simulink model "active_vehicle_ESP_Control"  (R2020a)
settings: Solver=ode4  StartTime=0.0  StopTime=inf  FixedStep=1e-3  RelTol=1e-3
InitFcn:
  | clear mex
model workspace (MAT data in the model file):
  inChnlList : object (value not decoded)
  inChnlListInternal : object (value not decoded)
  outChnlList : object (value not decoded)
  outChnlListInternal : object (value not decoded)
undefined symbols (not defined in the file or in its folder): DiscIntNeverNeededParam, vicrt_initcallback, vicrt_initmexcallback, vicrt_inputfile, vicrt_simulationmanager
libraries: simulink x1
(part 5 of 6)

== system active_vehicle_ESP_Control/Driveline/Engine/Engine Maps/Rpm control/idle control ==
  engine omega : Inport
  idle speed : Inport  Port=2
  Add2 : Sum  Inputs=+-  OutDataTypeStr=Inherit: Same as first input
  Gain : Gain  Gain=100*0.005/((2*pi/60))  OutDataTypeStr=Inherit: Same as input  ParamDataTypeStr=Inherit: Same as input
  Switch : Switch  Criteria=u2 > Threshold
  Unary Minus : UnaryMinus
  zero : Constant  Value=0
  rpm_idle_contrlol : Outport
  wires:
  engine omega/1 -> Add2/1
  idle speed/1 -> Add2/2
  Add2/1 -> Switch/2, Unary Minus/1
  zero/1 -> Switch/1
  Unary Minus/1 -> Gain/1
  Gain/1 -> Switch/3
  Switch/1 -> rpm_idle_contrlol/1

== system active_vehicle_ESP_Control/Vehicle/VI-CarRealTime/Input_Bus/Inputs/ABS ==
  ABS_threshold_def_val : Constant  Value=0
  BCABS : BusCreator  Inputs=2
  Internal_ABS_Activity_def_val : Constant
  ABS : Outport
  wires:
  BCABS/1 -> ABS/1  "ABS"
  Internal_ABS_Activity_def_val/1 -> BCABS/1  "Internal_ABS_Activity"
  ABS_threshold_def_val/1 -> BCABS/2  "ABS_threshold"

== system active_vehicle_ESP_Control/Vehicle/VI-CarRealTime/Input_Bus/Inputs/Aerodynamic ==
  BCAerodynamic : BusCreator  Inputs=16
  fx_center_def_val : Constant  Value=0
  fx_central_scaling_def_val : Constant
  fx_front_def_val : Constant  Value=0
  fx_rear_def_val : Constant  Value=0
  fy_center_def_val : Constant  Value=0
  fy_front_def_val : Constant  Value=0
  fy_rear_def_val : Constant  Value=0
  fz_center_def_val : Constant  Value=0
  fz_front_def_val : Constant  Value=0
  fz_front_scaling_def_val : Constant
  fz_rear_def_val : Constant  Value=0
  fz_rear_scaling_def_val : Constant
  mx_def_val : Constant  Value=0
  my_def_val : Constant  Value=0
  my_scaling_def_val : Constant
  mz_def_val : Constant  Value=0
  Aerodynamic : Outport
  wires:
  BCAerodynamic/1 -> Aerodynamic/1  "Aerodynamic"
  my_scaling_def_val/1 -> BCAerodynamic/1  "my_scaling"
  fx_central_scaling_def_val/1 -> BCAerodynamic/2  "fx_central_scaling"
  fz_front_scaling_def_val/1 -> BCAerodynamic/3  "fz_front_scaling"
  fz_rear_scaling_def_val/1 -> BCAerodynamic/4  "fz_rear_scaling"
  fx_front_def_val/1 -> BCAerodynamic/5  "fx_front"
  fy_front_def_val/1 -> BCAerodynamic/6  "fy_front"
  fz_front_def_val/1 -> BCAerodynamic/7  "fz_front"
  fx_rear_def_val/1 -> BCAerodynamic/8  "fx_rear"
  fy_rear_def_val/1 -> BCAerodynamic/9  "fy_rear"
  fz_rear_def_val/1 -> BCAerodynamic/10  "fz_rear"
  fx_center_def_val/1 -> BCAerodynamic/11  "fx_center"
  fy_center_def_val/1 -> BCAerodynamic/12  "fy_center"
  fz_center_def_val/1 -> BCAerodynamic/13  "fz_center"
  mx_def_val/1 -> BCAerodynamic/14  "mx"
  my_def_val/1 -> BCAerodynamic/15  "my"
  mz_def_val/1 -> BCAerodynamic/16  "mz"

== system active_vehicle_ESP_Control/Vehicle/VI-CarRealTime/Input_Bus/Inputs/Antiroll_Bar ==
  BCAntiroll_Bar : BusCreator  Inputs=2
  activity_flag : Subsystem
  force : Subsystem
  Antiroll_Bar : Outport
  wires:
  BCAntiroll_Bar/1 -> Antiroll_Bar/1  "Antiroll_Bar"
  activity_flag/1(activity_flag) -> BCAntiroll_Bar/1  "activity_flag"
  force/1(force) -> BCAntiroll_Bar/2  "force"

== system active_vehicle_ESP_Control/Vehicle/VI-CarRealTime/Input_Bus/Inputs/Auxiliary_vertical ==
  BCAuxiliary_vertical : BusCreator  Inputs=2
  activity_flag : Subsystem
  force : Subsystem
  Auxiliary_vertical : Outport
  wires:
  BCAuxiliary_vertical/1 -> Auxiliary_vertical/1  "Auxiliary_vertical"
  force/1(force) -> BCAuxiliary_vertical/1  "force"
  activity_flag/1(activity_flag) -> BCAuxiliary_vertical/2  "activity_flag"

== system active_vehicle_ESP_Control/Vehicle/VI-CarRealTime/Input_Bus/Inputs/Brake_System ==
  BCBrake_System : BusCreator  Inputs=5
  brk_mmag_sign : Subsystem
  brk_mmag_unsign : Subsystem
  brk_mu : Subsystem
  brk_pres : Subsystem
  brk_pres_gain : Subsystem
  Brake_System : Outport
  wires:
  BCBrake_System/1 -> Brake_System/1  "Brake_System"
  brk_mmag_sign/1(brk_mmag_sign) -> BCBrake_System/1  "brk_mmag_sign"
  brk_mmag_unsign/1(brk_mmag_unsign) -> BCBrake_System/2  "brk_mmag_unsign"
  brk_pres/1(brk_pres) -> BCBrake_System/3  "brk_pres"
  brk_pres_gain/1(brk_pres_gain) -> BCBrake_System/4  "brk_pres_gain"
  brk_mu/1(brk_mu) -> BCBrake_System/5  "brk_mu"

== system active_vehicle_ESP_Control/Vehicle/VI-CarRealTime/Input_Bus/Inputs/Brake_System_General ==
  BCBrake_System_General : BusCreator  Inputs=2
  brk_bias_front_def_val : Constant  Value=0
  brk_mast_cyl_pres_def_val : Constant  Value=0
  Brake_System_General : Outport
  wires:
  BCBrake_System_General/1 -> Brake_System_General/1  "Brake_System_General"
  brk_mast_cyl_pres_def_val/1 -> BCBrake_System_General/1  "brk_mast_cyl_pres"
  brk_bias_front_def_val/1 -> BCBrake_System_General/2  "brk_bias_front"

== system active_vehicle_ESP_Control/Vehicle/VI-CarRealTime/Input_Bus/Inputs/Clutch ==
  BCClutch : BusCreator  Inputs=6
  clutch_trq_def_val : Constant  Value=0
  efficiency_def_val : Constant
  gearbox_inputshaft_torque_def_val : Constant  Value=0
  inputplate_alpha_def_val : Constant  Value=-9999999
  inputplate_angle_def_val : Constant  Value=-9999999
  inputplate_omega_def_val : Constant  Value=-9999999
  Clutch : Outport
  wires:
  BCClutch/1 -> Clutch/1  "Clutch"
  clutch_trq_def_val/1 -> BCClutch/1  "clutch_trq"
  gearbox_inputshaft_torque_def_val/1 -> BCClutch/2  "gearbox_inputshaft_torque"
  inputplate_angle_def_val/1 -> BCClutch/3  "inputplate_angle"
  inputplate_omega_def_val/1 -> BCClutch/4  "inputplate_omega"
  inputplate_alpha_def_val/1 -> BCClutch/5  "inputplate_alpha"
  efficiency_def_val/1 -> BCClutch/6  "efficiency"

== system active_vehicle_ESP_Control/Vehicle/VI-CarRealTime/Input_Bus/Inputs/Differential_Central ==
  BCDifferential_Central : BusCreator  Inputs=6
  diff_front_inputshaft_torque_def_val : Constant  Value=0
  diff_rear_inputshaft_torque_def_val : Constant  Value=0
  efficiency_def_val : Constant
  gearbox_outputshaft_alpha_def_val : Constant  Value=0
  gearbox_outputshaft_angle_def_val : Constant  Value=0
  gearbox_outputshaft_omega_def_val : Constant  Value=0
  Differential_Central : Outport
  wires:
  BCDifferential_Central/1 -> Differential_Central/1  "Differential_Central"
  efficiency_def_val/1 -> BCDifferential_Central/1  "efficiency"
  diff_front_inputshaft_torque_def_val/1 -> BCDifferential_Central/2  "diff_front_inputshaft_torque"
  diff_rear_inputshaft_torque_def_val/1 -> BCDifferential_Central/3  "diff_rear_inputshaft_torque"
  gearbox_outputshaft_angle_def_val/1 -> BCDifferential_Central/4  "gearbox_outputshaft_angle"
  gearbox_outputshaft_omega_def_val/1 -> BCDifferential_Central/5  "gearbox_outputshaft_omega"
  gearbox_outputshaft_alpha_def_val/1 -> BCDifferential_Central/6  "gearbox_outputshaft_alpha"

== system active_vehicle_ESP_Control/Vehicle/VI-CarRealTime/Input_Bus/Inputs/Differential_Front ==
  BCDifferential_Front : BusCreator  Inputs=6
  diff_central_front_outputshaft_alpha_def_val : Constant  Value=0
  diff_central_front_outputshaft_angle_def_val : Constant  Value=0
  diff_central_front_outputshaft_omega_def_val : Constant  Value=0
  efficiency_def_val : Constant
  wheel_front_left_torque_def_val : Constant  Value=0
  wheel_front_right_torque_def_val : Constant  Value=0
  Differential_Front : Outport
  wires:
  BCDifferential_Front/1 -> Differential_Front/1  "Differential_Front"
  efficiency_def_val/1 -> BCDifferential_Front/1  "efficiency"
  wheel_front_left_torque_def_val/1 -> BCDifferential_Front/2  "wheel_front_left_torque"
  wheel_front_right_torque_def_val/1 -> BCDifferential_Front/3  "wheel_front_right_torque"
  diff_central_front_outputshaft_angle_def_val/1 -> BCDifferential_Front/4  "diff_central_front_outputshaft_angle"
  diff_central_front_outputshaft_omega_def_val/1 -> BCDifferential_Front/5  "diff_central_front_outputshaft_omega"
  diff_central_front_outputshaft_alpha_def_val/1 -> BCDifferential_Front/6  "diff_central_front_outputshaft_alpha"

== system active_vehicle_ESP_Control/Vehicle/VI-CarRealTime/Input_Bus/Inputs/Differential_Rear ==
  BCDifferential_Rear : BusCreator  Inputs=6
  diff_central_rear_outputshaft_alpha_def_val : Constant  Value=0
  diff_central_rear_outputshaft_angle_def_val : Constant  Value=0
  diff_central_rear_outputshaft_omega_def_val : Constant  Value=0
  efficiency_def_val : Constant
  wheel_rear_left_torque_def_val : Constant  Value=0
  wheel_rear_right_torque_def_val : Constant  Value=0
  Differential_Rear : Outport
  wires:
  BCDifferential_Rear/1 -> Differential_Rear/1  "Differential_Rear"
  efficiency_def_val/1 -> BCDifferential_Rear/1  "efficiency"
  wheel_rear_left_torque_def_val/1 -> BCDifferential_Rear/2  "wheel_rear_left_torque"
  wheel_rear_right_torque_def_val/1 -> BCDifferential_Rear/3  "wheel_rear_right_torque"
  diff_central_rear_outputshaft_angle_def_val/1 -> BCDifferential_Rear/4  "diff_central_rear_outputshaft_angle"
  diff_central_rear_outputshaft_omega_def_val/1 -> BCDifferential_Rear/5  "diff_central_rear_outputshaft_omega"
  diff_central_rear_outputshaft_alpha_def_val/1 -> BCDifferential_Rear/6  "diff_central_rear_outputshaft_alpha"

== system active_vehicle_ESP_Control/Vehicle/VI-CarRealTime/Input_Bus/Inputs/Driver_Demands ==
  BCDriver_Demands : BusCreator  Inputs=14
  brake_def_val : Constant  Value=0
  clutch_def_val : Constant  Value=0
  gear_def_val : Constant  Value=0
  rack_displacement_def_val : Constant  Value=0
  str_swa_def_val : Constant  Value=0
  target_acc_def_val : Constant  Value=0
  target_speed_def_val : Constant  Value=0
  throttle_def_val : Constant  Value=0
  user_input_braking_def_val : Constant  Value=0
  user_input_clutch_def_val : Constant  Value=0
  user_input_gear_def_val : Constant  Value=0
  user_input_steering_def_val : Constant  Value=0
  user_input_throttle_def_val : Constant  Value=0
  user_maneuver_ID_def_val : Constant  Value=0
  Driver_Demands : Outport
  wires:
  BCDriver_Demands/1 -> Driver_Demands/1  "Driver_Demands"
  str_swa_def_val/1 -> BCDriver_Demands/1  "str_swa"
  rack_displacement_def_val/1 -> BCDriver_Demands/2  "rack_displacement"
  throttle_def_val/1 -> BCDriver_Demands/3  "throttle"
  gear_def_val/1 -> BCDriver_Demands/4  "gear"
  clutch_def_val/1 -> BCDriver_Demands/5  "clutch"
  brake_def_val/1 -> BCDriver_Demands/6  "brake"
  target_speed_def_val/1 -> BCDriver_Demands/7  "target_speed"
  target_acc_def_val/1 -> BCDriver_Demands/8  "target_acc"
  user_maneuver_ID_def_val/1 -> BCDriver_Demands/9  "user_maneuver_ID"
  user_input_steering_def_val/1 -> BCDriver_Demands/10  "user_input_steering"
  user_input_throttle_def_val/1 -> BCDriver_Demands/11  "user_input_throttle"
  user_input_braking_def_val/1 -> BCDriver_Demands/12  "user_input_braking"
  user_input_gear_def_val/1 -> BCDriver_Demands/13  "user_input_gear"
  user_input_clutch_def_val/1 -> BCDriver_Demands/14  "user_input_clutch"

== system active_vehicle_ESP_Control/Vehicle/VI-CarRealTime/Input_Bus/Inputs/Engine ==
  BCEngine : BusCreator  Inputs=10
  clutch_inputplate_torque_def_val : Constant  Value=0
  control_mode_def_val : Constant
  efficiency_def_val : Constant
  engine_max_trq_def_val : Constant  Value=0
  engine_min_trq_def_val : Constant  Value=0
  engine_omega_def_val : Constant  Value=0
  engine_trq_def_val : Constant  Value=0
  non_termic_engine_trq_def_val : Constant  Value=0
  throttle_offset_def_val : Constant  Value=0
  throttle_scaling_def_val : Constant
  Engine : Outport
  wires:
  BCEngine/1 -> Engine/1  "Engine"
  engine_omega_def_val/1 -> BCEngine/1  "engine_omega"
  engine_max_trq_def_val/1 -> BCEngine/2  "engine_max_trq"
  engine_min_trq_def_val/1 -> BCEngine/3  "engine_min_trq"
  engine_trq_def_val/1 -> BCEngine/4  "engine_trq"
  clutch_inputplate_torque_def_val/1 -> BCEngine/5  "clutch_inputplate_torque"
  non_termic_engine_trq_def_val/1 -> BCEngine/6  "non_termic_engine_trq"
  efficiency_def_val/1 -> BCEngine/7  "efficiency"
  throttle_scaling_def_val/1 -> BCEngine/8  "throttle_scaling"
  control_mode_def_val/1 -> BCEngine/9  "control_mode"
  throttle_offset_def_val/1 -> BCEngine/10  "throttle_offset"

== system active_vehicle_ESP_Control/Vehicle/VI-CarRealTime/Input_Bus/Inputs/Ext_Body ==
  BCExt_Body : BusCreator  Inputs=2
  force : Subsystem
  moment : Subsystem
  Ext_Body : Outport
  wires:
  BCExt_Body/1 -> Ext_Body/1  "Ext_Body"
  force/1(force) -> BCExt_Body/1  "force"
  moment/1(moment) -> BCExt_Body/2  "moment"

== system active_vehicle_ESP_Control/Vehicle/VI-CarRealTime/Input_Bus/Inputs/Ext_Ground ==
  BCExt_Ground : BusCreator  Inputs=2
  force : Subsystem
  moment : Subsystem
  Ext_Ground : Outport
  wires:
  BCExt_Ground/1 -> Ext_Ground/1  "Ext_Ground"
  force/1(force) -> BCExt_Ground/1  "force"
  moment/1(moment) -> BCExt_Ground/2  "moment"

== system active_vehicle_ESP_Control/Vehicle/VI-CarRealTime/Input_Bus/Inputs/Ext_Tracking ==
  BCExt_Tracking : BusCreator  Inputs=2
  force : Subsystem
  moment : Subsystem
  Ext_Tracking : Outport
  wires:
  BCExt_Tracking/1 -> Ext_Tracking/1  "Ext_Tracking"
  force/1(force) -> BCExt_Tracking/1  "force"
  moment/1(moment) -> BCExt_Tracking/2  "moment"

== system active_vehicle_ESP_Control/Vehicle/VI-CarRealTime/Input_Bus/Inputs/Friction ==
  BCFriction : BusCreator  Inputs=1
  tire_mu : Subsystem
  Friction : Outport
  wires:
  BCFriction/1 -> Friction/1  "Friction"
  tire_mu/1(tire_mu) -> BCFriction/1  "tire_mu"

== system active_vehicle_ESP_Control/Vehicle/VI-CarRealTime/Input_Bus/Inputs/GearBox ==
  BCGearBox : BusCreator  Inputs=7
  automatic_gearbox_shifting_mode_def_val : Constant  Value=-9999999
  clutch_outputplate_alpha_def_val : Constant  Value=-9999999
  clutch_outputplate_angle_def_val : Constant  Value=-9999999
  clutch_outputplate_omega_def_val : Constant  Value=-9999999
  diff_central_inputshaft_torque_def_val : Constant  Value=0
  efficiency_def_val : Constant
  transmission_ratio_def_val : Constant  Value=0
  GearBox : Outport
  wires:
  BCGearBox/1 -> GearBox/1  "GearBox"
  efficiency_def_val/1 -> BCGearBox/1  "efficiency"
  transmission_ratio_def_val/1 -> BCGearBox/2  "transmission_ratio"
  diff_central_inputshaft_torque_def_val/1 -> BCGearBox/3  "diff_central_inputshaft_torque"
  clutch_outputplate_angle_def_val/1 -> BCGearBox/4  "clutch_outputplate_angle"
  clutch_outputplate_omega_def_val/1 -> BCGearBox/5  "clutch_outputplate_omega"
  clutch_outputplate_alpha_def_val/1 -> BCGearBox/6  "clutch_outputplate_alpha"
  automatic_gearbox_shifting_mode_def_val/1 -> BCGearBox/7  "automatic_gearbox_shifting_mode"

== system active_vehicle_ESP_Control/Vehicle/VI-CarRealTime/Input_Bus/Inputs/Generic_Engine_to_Central_Differential ==
  BCGeneric_Engine_to_Central_Differential : BusCreator  Inputs=10
  control_mode_def_val : Constant
  efficiency_def_val : Constant
  engine_max_torque_def_val : Constant  Value=0
  engine_min_torque_def_val : Constant  Value=0
  engine_torque_def_val : Constant  Value=0
  regeneration_factor_def_val : Constant
  reverse_mode_def_val : Constant  Value=0
  throttle_offset_def_val : Constant  Value=0
  throttle_scaling_def_val : Constant
  transmission_ratio_def_val : Constant
  Generic_Engine_to_Central_Differential : Outport
  wires:
  BCGeneric_Engine_to_Central_Differential/1 -> Generic_Engine_to_Central_Differential/1  "Generic_Engine_to_Central_Differential"
  transmission_ratio_def_val/1 -> BCGeneric_Engine_to_Central_Differential/1  "transmission_ratio"
  reverse_mode_def_val/1 -> BCGeneric_Engine_to_Central_Differential/2  "reverse_mode"
  regeneration_factor_def_val/1 -> BCGeneric_Engine_to_Central_Differential/3  "regeneration_factor"
  throttle_scaling_def_val/1 -> BCGeneric_Engine_to_Central_Differential/4  "throttle_scaling"
  control_mode_def_val/1 -> BCGeneric_Engine_to_Central_Differential/5  "control_mode"
  throttle_offset_def_val/1 -> BCGeneric_Engine_to_Central_Differential/6  "throttle_offset"
  efficiency_def_val/1 -> BCGeneric_Engine_to_Central_Differential/7  "efficiency"
  engine_torque_def_val/1 -> BCGeneric_Engine_to_Central_Differential/8  "engine_torque"
  engine_max_torque_def_val/1 -> BCGeneric_Engine_to_Central_Differential/9  "engine_max_torque"
  engine_min_torque_def_val/1 -> BCGeneric_Engine_to_Central_Differential/10  "engine_min_torque"

== system active_vehicle_ESP_Control/Vehicle/VI-CarRealTime/Input_Bus/Inputs/Generic_Engine_to_Clutch ==
  BCGeneric_Engine_to_Clutch : BusCreator  Inputs=9
  control_mode_def_val : Constant
  efficiency_def_val : Constant
  engine_max_torque_def_val : Constant  Value=0
  engine_min_torque_def_val : Constant  Value=0
  engine_torque_def_val : Constant  Value=0
  regeneration_factor_def_val : Constant
  throttle_offset_def_val : Constant  Value=0
  throttle_scaling_def_val : Constant
  transmission_ratio_def_val : Constant
  Generic_Engine_to_Clutch : Outport
  wires:
  BCGeneric_Engine_to_Clutch/1 -> Generic_Engine_to_Clutch/1  "Generic_Engine_to_Clutch"
  transmission_ratio_def_val/1 -> BCGeneric_Engine_to_Clutch/1  "transmission_ratio"
  regeneration_factor_def_val/1 -> BCGeneric_Engine_to_Clutch/2  "regeneration_factor"
  throttle_scaling_def_val/1 -> BCGeneric_Engine_to_Clutch/3  "throttle_scaling"
  control_mode_def_val/1 -> BCGeneric_Engine_to_Clutch/4  "control_mode"
  throttle_offset_def_val/1 -> BCGeneric_Engine_to_Clutch/5  "throttle_offset"
  efficiency_def_val/1 -> BCGeneric_Engine_to_Clutch/6  "efficiency"
  engine_torque_def_val/1 -> BCGeneric_Engine_to_Clutch/7  "engine_torque"
  engine_max_torque_def_val/1 -> BCGeneric_Engine_to_Clutch/8  "engine_max_torque"
  engine_min_torque_def_val/1 -> BCGeneric_Engine_to_Clutch/9  "engine_min_torque"

== system active_vehicle_ESP_Control/Vehicle/VI-CarRealTime/Input_Bus/Inputs/Generic_Engine_to_Front_Differential ==
  BCGeneric_Engine_to_Front_Differential : BusCreator  Inputs=10
  control_mode_def_val : Constant
  efficiency_def_val : Constant
  engine_max_torque_def_val : Constant  Value=0
  engine_min_torque_def_val : Constant  Value=0
  engine_torque_def_val : Constant  Value=0
  regeneration_factor_def_val : Constant
  reverse_mode_def_val : Constant  Value=0
  throttle_offset_def_val : Constant  Value=0
  throttle_scaling_def_val : Constant
  transmission_ratio_def_val : Constant
  Generic_Engine_to_Front_Differential : Outport
  wires:
  BCGeneric_Engine_to_Front_Differential/1 -> Generic_Engine_to_Front_Differential/1  "Generic_Engine_to_Front_Differential"
  transmission_ratio_def_val/1 -> BCGeneric_Engine_to_Front_Differential/1  "transmission_ratio"
  reverse_mode_def_val/1 -> BCGeneric_Engine_to_Front_Differential/2  "reverse_mode"
  regeneration_factor_def_val/1 -> BCGeneric_Engine_to_Front_Differential/3  "regeneration_factor"
  throttle_scaling_def_val/1 -> BCGeneric_Engine_to_Front_Differential/4  "throttle_scaling"
  control_mode_def_val/1 -> BCGeneric_Engine_to_Front_Differential/5  "control_mode"
  throttle_offset_def_val/1 -> BCGeneric_Engine_to_Front_Differential/6  "throttle_offset"
  efficiency_def_val/1 -> BCGeneric_Engine_to_Front_Differential/7  "efficiency"
  engine_torque_def_val/1 -> BCGeneric_Engine_to_Front_Differential/8  "engine_torque"
  engine_max_torque_def_val/1 -> BCGeneric_Engine_to_Front_Differential/9  "engine_max_torque"
  engine_min_torque_def_val/1 -> BCGeneric_Engine_to_Front_Differential/10  "engine_min_torque"

== system active_vehicle_ESP_Control/Vehicle/VI-CarRealTime/Input_Bus/Inputs/Generic_Engine_to_Front_Left_Wheel ==
  BCGeneric_Engine_to_Front_Left_Wheel : BusCreator  Inputs=10
  control_mode_def_val : Constant
  efficiency_def_val : Constant
  engine_max_torque_def_val : Constant  Value=0
  engine_min_torque_def_val : Constant  Value=0
  engine_torque_def_val : Constant  Value=0
  regeneration_factor_def_val : Constant
  reverse_mode_def_val : Constant  Value=0
  throttle_offset_def_val : Constant  Value=0
  throttle_scaling_def_val : Constant
  transmission_ratio_def_val : Constant
  Generic_Engine_to_Front_Left_Wheel : Outport
  wires:
  BCGeneric_Engine_to_Front_Left_Wheel/1 -> Generic_Engine_to_Front_Left_Wheel/1  "Generic_Engine_to_Front_Left_Wheel"
  transmission_ratio_def_val/1 -> BCGeneric_Engine_to_Front_Left_Wheel/1  "transmission_ratio"
  reverse_mode_def_val/1 -> BCGeneric_Engine_to_Front_Left_Wheel/2  "reverse_mode"
  regeneration_factor_def_val/1 -> BCGeneric_Engine_to_Front_Left_Wheel/3  "regeneration_factor"
  throttle_scaling_def_val/1 -> BCGeneric_Engine_to_Front_Left_Wheel/4  "throttle_scaling"
  control_mode_def_val/1 -> BCGeneric_Engine_to_Front_Left_Wheel/5  "control_mode"
  throttle_offset_def_val/1 -> BCGeneric_Engine_to_Front_Left_Wheel/6  "throttle_offset"
  efficiency_def_val/1 -> BCGeneric_Engine_to_Front_Left_Wheel/7  "efficiency"
  engine_torque_def_val/1 -> BCGeneric_Engine_to_Front_Left_Wheel/8  "engine_torque"
  engine_max_torque_def_val/1 -> BCGeneric_Engine_to_Front_Left_Wheel/9  "engine_max_torque"
  engine_min_torque_def_val/1 -> BCGeneric_Engine_to_Front_Left_Wheel/10  "engine_min_torque"

== system active_vehicle_ESP_Control/Vehicle/VI-CarRealTime/Input_Bus/Inputs/Generic_Engine_to_Front_Right_Wheel ==
  BCGeneric_Engine_to_Front_Right_Wheel : BusCreator  Inputs=10
  control_mode_def_val : Constant
  efficiency_def_val : Constant
  engine_max_torque_def_val : Constant  Value=0
  engine_min_torque_def_val : Constant  Value=0
  engine_torque_def_val : Constant  Value=0
  regeneration_factor_def_val : Constant
  reverse_mode_def_val : Constant  Value=0
  throttle_offset_def_val : Constant  Value=0
  throttle_scaling_def_val : Constant
  transmission_ratio_def_val : Constant
  Generic_Engine_to_Front_Right_Wheel : Outport
  wires:
  BCGeneric_Engine_to_Front_Right_Wheel/1 -> Generic_Engine_to_Front_Right_Wheel/1  "Generic_Engine_to_Front_Right_Wheel"
  transmission_ratio_def_val/1 -> BCGeneric_Engine_to_Front_Right_Wheel/1  "transmission_ratio"
  reverse_mode_def_val/1 -> BCGeneric_Engine_to_Front_Right_Wheel/2  "reverse_mode"
  regeneration_factor_def_val/1 -> BCGeneric_Engine_to_Front_Right_Wheel/3  "regeneration_factor"
  throttle_scaling_def_val/1 -> BCGeneric_Engine_to_Front_Right_Wheel/4  "throttle_scaling"
  control_mode_def_val/1 -> BCGeneric_Engine_to_Front_Right_Wheel/5  "control_mode"
  throttle_offset_def_val/1 -> BCGeneric_Engine_to_Front_Right_Wheel/6  "throttle_offset"
  efficiency_def_val/1 -> BCGeneric_Engine_to_Front_Right_Wheel/7  "efficiency"
  engine_torque_def_val/1 -> BCGeneric_Engine_to_Front_Right_Wheel/8  "engine_torque"
  engine_max_torque_def_val/1 -> BCGeneric_Engine_to_Front_Right_Wheel/9  "engine_max_torque"
  engine_min_torque_def_val/1 -> BCGeneric_Engine_to_Front_Right_Wheel/10  "engine_min_torque"

== system active_vehicle_ESP_Control/Vehicle/VI-CarRealTime/Input_Bus/Inputs/Generic_Engine_to_Gearbox ==
  BCGeneric_Engine_to_Gearbox : BusCreator  Inputs=9
  control_mode_def_val : Constant
  efficiency_def_val : Constant
  engine_max_torque_def_val : Constant  Value=0
  engine_min_torque_def_val : Constant  Value=0
  engine_torque_def_val : Constant  Value=0
  regeneration_factor_def_val : Constant
  throttle_offset_def_val : Constant  Value=0
  throttle_scaling_def_val : Constant
  transmission_ratio_def_val : Constant
  Generic_Engine_to_Gearbox : Outport
  wires:
  BCGeneric_Engine_to_Gearbox/1 -> Generic_Engine_to_Gearbox/1  "Generic_Engine_to_Gearbox"
  transmission_ratio_def_val/1 -> BCGeneric_Engine_to_Gearbox/1  "transmission_ratio"
  regeneration_factor_def_val/1 -> BCGeneric_Engine_to_Gearbox/2  "regeneration_factor"
  throttle_scaling_def_val/1 -> BCGeneric_Engine_to_Gearbox/3  "throttle_scaling"
  control_mode_def_val/1 -> BCGeneric_Engine_to_Gearbox/4  "control_mode"
  throttle_offset_def_val/1 -> BCGeneric_Engine_to_Gearbox/5  "throttle_offset"
  efficiency_def_val/1 -> BCGeneric_Engine_to_Gearbox/6  "efficiency"
  engine_torque_def_val/1 -> BCGeneric_Engine_to_Gearbox/7  "engine_torque"
  engine_max_torque_def_val/1 -> BCGeneric_Engine_to_Gearbox/8  "engine_max_torque"
  engine_min_torque_def_val/1 -> BCGeneric_Engine_to_Gearbox/9  "engine_min_torque"

== system active_vehicle_ESP_Control/Vehicle/VI-CarRealTime/Input_Bus/Inputs/Generic_Engine_to_Rear_Differential ==
  BCGeneric_Engine_to_Rear_Differential : BusCreator  Inputs=10
  control_mode_def_val : Constant
  efficiency_def_val : Constant
  engine_max_torque_def_val : Constant  Value=0
  engine_min_torque_def_val : Constant  Value=0
  engine_torque_def_val : Constant  Value=0
  regeneration_factor_def_val : Constant
  reverse_mode_def_val : Constant  Value=0
  throttle_offset_def_val : Constant  Value=0
  throttle_scaling_def_val : Constant
  transmission_ratio_def_val : Constant
  Generic_Engine_to_Rear_Differential : Outport
  wires:
  BCGeneric_Engine_to_Rear_Differential/1 -> Generic_Engine_to_Rear_Differential/1  "Generic_Engine_to_Rear_Differential"
  transmission_ratio_def_val/1 -> BCGeneric_Engine_to_Rear_Differential/1  "transmission_ratio"
  reverse_mode_def_val/1 -> BCGeneric_Engine_to_Rear_Differential/2  "reverse_mode"
  regeneration_factor_def_val/1 -> BCGeneric_Engine_to_Rear_Differential/3  "regeneration_factor"
  throttle_scaling_def_val/1 -> BCGeneric_Engine_to_Rear_Differential/4  "throttle_scaling"
  control_mode_def_val/1 -> BCGeneric_Engine_to_Rear_Differential/5  "control_mode"
  throttle_offset_def_val/1 -> BCGeneric_Engine_to_Rear_Differential/6  "throttle_offset"
  efficiency_def_val/1 -> BCGeneric_Engine_to_Rear_Differential/7  "efficiency"
  engine_torque_def_val/1 -> BCGeneric_Engine_to_Rear_Differential/8  "engine_torque"
  engine_max_torque_def_val/1 -> BCGeneric_Engine_to_Rear_Differential/9  "engine_max_torque"
  engine_min_torque_def_val/1 -> BCGeneric_Engine_to_Rear_Differential/10  "engine_min_torque"

== system active_vehicle_ESP_Control/Vehicle/VI-CarRealTime/Input_Bus/Inputs/Generic_Engine_to_Rear_Left_Wheel ==
  BCGeneric_Engine_to_Rear_Left_Wheel : BusCreator  Inputs=10
  control_mode_def_val : Constant
  efficiency_def_val : Constant
  engine_max_torque_def_val : Constant  Value=0
  engine_min_torque_def_val : Constant  Value=0
  engine_torque_def_val : Constant  Value=0
  regeneration_factor_def_val : Constant
  reverse_mode_def_val : Constant  Value=0
  throttle_offset_def_val : Constant  Value=0
  throttle_scaling_def_val : Constant
  transmission_ratio_def_val : Constant
  Generic_Engine_to_Rear_Left_Wheel : Outport
  wires:
  BCGeneric_Engine_to_Rear_Left_Wheel/1 -> Generic_Engine_to_Rear_Left_Wheel/1  "Generic_Engine_to_Rear_Left_Wheel"
  transmission_ratio_def_val/1 -> BCGeneric_Engine_to_Rear_Left_Wheel/1  "transmission_ratio"
  reverse_mode_def_val/1 -> BCGeneric_Engine_to_Rear_Left_Wheel/2  "reverse_mode"
  regeneration_factor_def_val/1 -> BCGeneric_Engine_to_Rear_Left_Wheel/3  "regeneration_factor"
  throttle_scaling_def_val/1 -> BCGeneric_Engine_to_Rear_Left_Wheel/4  "throttle_scaling"
  control_mode_def_val/1 -> BCGeneric_Engine_to_Rear_Left_Wheel/5  "control_mode"
  throttle_offset_def_val/1 -> BCGeneric_Engine_to_Rear_Left_Wheel/6  "throttle_offset"
  efficiency_def_val/1 -> BCGeneric_Engine_to_Rear_Left_Wheel/7  "efficiency"
  engine_torque_def_val/1 -> BCGeneric_Engine_to_Rear_Left_Wheel/8  "engine_torque"
  engine_max_torque_def_val/1 -> BCGeneric_Engine_to_Rear_Left_Wheel/9  "engine_max_torque"
  engine_min_torque_def_val/1 -> BCGeneric_Engine_to_Rear_Left_Wheel/10  "engine_min_torque"

== system active_vehicle_ESP_Control/Vehicle/VI-CarRealTime/Input_Bus/Inputs/Generic_Engine_to_Rear_Right_Wheel ==
  BCGeneric_Engine_to_Rear_Right_Wheel : BusCreator  Inputs=10
  control_mode_def_val : Constant
  efficiency_def_val : Constant
  engine_max_torque_def_val : Constant  Value=0
  engine_min_torque_def_val : Constant  Value=0
  engine_torque_def_val : Constant  Value=0
  regeneration_factor_def_val : Constant
  reverse_mode_def_val : Constant  Value=0
  throttle_offset_def_val : Constant  Value=0
  throttle_scaling_def_val : Constant
  transmission_ratio_def_val : Constant
  Generic_Engine_to_Rear_Right_Wheel : Outport
  wires:
  BCGeneric_Engine_to_Rear_Right_Wheel/1 -> Generic_Engine_to_Rear_Right_Wheel/1  "Generic_Engine_to_Rear_Right_Wheel"
  transmission_ratio_def_val/1 -> BCGeneric_Engine_to_Rear_Right_Wheel/1  "transmission_ratio"
  reverse_mode_def_val/1 -> BCGeneric_Engine_to_Rear_Right_Wheel/2  "reverse_mode"
  regeneration_factor_def_val/1 -> BCGeneric_Engine_to_Rear_Right_Wheel/3  "regeneration_factor"
  throttle_scaling_def_val/1 -> BCGeneric_Engine_to_Rear_Right_Wheel/4  "throttle_scaling"
  control_mode_def_val/1 -> BCGeneric_Engine_to_Rear_Right_Wheel/5  "control_mode"
  throttle_offset_def_val/1 -> BCGeneric_Engine_to_Rear_Right_Wheel/6  "throttle_offset"
  efficiency_def_val/1 -> BCGeneric_Engine_to_Rear_Right_Wheel/7  "efficiency"
  engine_torque_def_val/1 -> BCGeneric_Engine_to_Rear_Right_Wheel/8  "engine_torque"
  engine_max_torque_def_val/1 -> BCGeneric_Engine_to_Rear_Right_Wheel/9  "engine_max_torque"
  engine_min_torque_def_val/1 -> BCGeneric_Engine_to_Rear_Right_Wheel/10  "engine_min_torque"

== system active_vehicle_ESP_Control/Vehicle/VI-CarRealTime/Input_Bus/Inputs/Hook ==
  BCHook : BusCreator  Inputs=6
  Fx : Subsystem
  Fy : Subsystem
  Fz : Subsystem
  Mx : Subsystem
  My : Subsystem
  Mz : Subsystem
  Hook : Outport
  wires:
  BCHook/1 -> Hook/1  "Hook"
  Fx/1(Fx) -> BCHook/1  "Fx"
  Fy/1(Fy) -> BCHook/2  "Fy"
  Fz/1(Fz) -> BCHook/3  "Fz"
  Mx/1(Mx) -> BCHook/4  "Mx"
  My/1(My) -> BCHook/5  "My"
  Mz/1(Mz) -> BCHook/6  "Mz"

== system active_vehicle_ESP_Control/Vehicle/VI-CarRealTime/Input_Bus/Inputs/Irregularity ==
  BCIrregularity : BusCreator  Inputs=1
  road : Subsystem
  Irregularity : Outport
  wires:
  BCIrregularity/1 -> Irregularity/1  "Irregularity"
  road/1(road) -> BCIrregularity/1  "road"

== system active_vehicle_ESP_Control/Vehicle/VI-CarRealTime/Input_Bus/Inputs/Main_Bumpstop ==
  BCMain_Bumpstop : BusCreator  Inputs=2
  activity_flag : Subsystem
  force : Subsystem
  Main_Bumpstop : Outport
  wires:
  BCMain_Bumpstop/1 -> Main_Bumpstop/1  "Main_Bumpstop"
  force/1(force) -> BCMain_Bumpstop/1  "force"
  activity_flag/1(activity_flag) -> BCMain_Bumpstop/2  "activity_flag"

== system active_vehicle_ESP_Control/Vehicle/VI-CarRealTime/Input_Bus/Inputs/Main_Damper ==
  BCMain_Damper : BusCreator  Inputs=2
  activity_flag : Subsystem
  force : Subsystem
  Main_Damper : Outport
  wires:
  BCMain_Damper/1 -> Main_Damper/1  "Main_Damper"
  force/1(force) -> BCMain_Damper/1  "force"
  activity_flag/1(activity_flag) -> BCMain_Damper/2  "activity_flag"

== system active_vehicle_ESP_Control/Vehicle/VI-CarRealTime/Input_Bus/Inputs/Main_Inerter ==
  BCMain_Inerter : BusCreator  Inputs=2
  activity_flag : Subsystem
  force : Subsystem
  Main_Inerter : Outport
  wires:
  BCMain_Inerter/1 -> Main_Inerter/1  "Main_Inerter"
  force/1(force) -> BCMain_Inerter/1  "force"
  activity_flag/1(activity_flag) -> BCMain_Inerter/2  "activity_flag"

== system active_vehicle_ESP_Control/Vehicle/VI-CarRealTime/Input_Bus/Inputs/Main_Reboundstop ==
  BCMain_Reboundstop : BusCreator  Inputs=2
  activity_flag : Subsystem
  force : Subsystem
  Main_Reboundstop : Outport
  wires:
  BCMain_Reboundstop/1 -> Main_Reboundstop/1  "Main_Reboundstop"
  force/1(force) -> BCMain_Reboundstop/1  "force"
  activity_flag/1(activity_flag) -> BCMain_Reboundstop/2  "activity_flag"

== system active_vehicle_ESP_Control/Vehicle/VI-CarRealTime/Input_Bus/Inputs/Main_Spring ==
  BCMain_Spring : BusCreator  Inputs=2
  activity_flag : Subsystem
  force : Subsystem
  Main_Spring : Outport
  wires:
  BCMain_Spring/1 -> Main_Spring/1  "Main_Spring"
  force/1(force) -> BCMain_Spring/1  "force"
  activity_flag/1(activity_flag) -> BCMain_Spring/2  "activity_flag"

== system active_vehicle_ESP_Control/Vehicle/VI-CarRealTime/Input_Bus/Inputs/Mono_Element ==
  BCMono_Element : BusCreator  Inputs=16
  Bumpstop_Damper : Subsystem
  Bumpstop_Damper_activity_flag : Subsystem
  Bumpstop_Spring : Subsystem
  Bumpstop_Spring_activity_flag : Subsystem
  Damper : Subsystem
  Damper_activity_flag : Subsystem
  Inerter : Subsystem
  Inerter_activity_flag : Subsystem
  Reboundstop_Damper : Subsystem
  Reboundstop_Damper_activity_flag : Subsystem
  Reboundstop_Spring : Subsystem
  Reboundstop_Spring_activity_flag : Subsystem
  Roll_Damper : Subsystem
  Roll_Damper_activity_flag : Subsystem
  Spring : Subsystem
  Spring_activity_flag : Subsystem
  Mono_Element : Outport
  wires:
  BCMono_Element/1 -> Mono_Element/1  "Mono_Element"
  Damper/1(Damper) -> BCMono_Element/1  "Damper"
  Damper_activity_flag/1(Damper_activity_flag) -> BCMono_Element/2  "Damper_activity_flag"
  Inerter/1(Inerter) -> BCMono_Element/3  "Inerter"
  Inerter_activity_flag/1(Inerter_activity_flag) -> BCMono_Element/4  "Inerter_activity_flag"
  Spring/1(Spring) -> BCMono_Element/5  "Spring"
  Spring_activity_flag/1(Spring_activity_flag) -> BCMono_Element/6  "Spring_activity_flag"
  Bumpstop_Spring/1(Bumpstop_Spring) -> BCMono_Element/7  "Bumpstop_Spring"
  Bumpstop_Spring_activity_flag/1(Bumpstop_Spring_activity_flag) -> BCMono_Element/8  "Bumpstop_Spring_activity_flag"
  Reboundstop_Spring/1(Reboundstop_Spring) -> BCMono_Element/9  "Reboundstop_Spring"
  Reboundstop_Spring_activity_flag/1(Reboundstop_Spring_activity_flag) -> BCMono_Element/10  "Reboundstop_Spring_activity_flag"
  Bumpstop_Damper/1(Bumpstop_Damper) -> BCMono_Element/11  "Bumpstop_Damper"
  Bumpstop_Damper_activity_flag/1(Bumpstop_Damper_activity_flag) -> BCMono_Element/12  "Bumpstop_Damper_activity_flag"
  Reboundstop_Damper/1(Reboundstop_Damper) -> BCMono_Element/13  "Reboundstop_Damper"
  Reboundstop_Damper_activity_flag/1(Reboundstop_Damper_activity_flag) -> BCMono_Element/14  "Reboundstop_Damper_activity_flag"
  Roll_Damper/1(Roll_Damper) -> BCMono_Element/15  "Roll_Damper"
  Roll_Damper_activity_flag/1(Roll_Damper_activity_flag) -> BCMono_Element/16  "Roll_Damper_activity_flag"

== system active_vehicle_ESP_Control/Vehicle/VI-CarRealTime/Input_Bus/Inputs/Rear_Steering_Actuator_disp ==
  BCRear_Steering_Actuator_disp : BusCreator  Inputs=1
  str_swa : Subsystem
  Rear_Steering_Actuator_disp : Outport
  wires:
  BCRear_Steering_Actuator_disp/1 -> Rear_Steering_Actuator_disp/1  "Rear_Steering_Actuator_disp"
  str_swa/1(str_swa) -> BCRear_Steering_Actuator_disp/1  "str_swa"

== system active_vehicle_ESP_Control/Vehicle/VI-CarRealTime/Input_Bus/Inputs/Steering ==
  BCSteering : BusCreator  Inputs=3
  Hand_Wheel_Torque_def_val : Constant  Value=0
  Internal_Hand_Wheel_Torque_Computation_def_val : Constant
  steer_at_spindle : Subsystem
  Steering : Outport
  wires:
  BCSteering/1 -> Steering/1  "Steering"
  steer_at_spindle/1(steer_at_spindle) -> BCSteering/1  "steer_at_spindle"
  Internal_Hand_Wheel_Torque_Computation_def_val/1 -> BCSteering/2  "Internal_Hand_Wheel_Torque_Computation"
  Hand_Wheel_Torque_def_val/1 -> BCSteering/3  "Hand_Wheel_Torque"

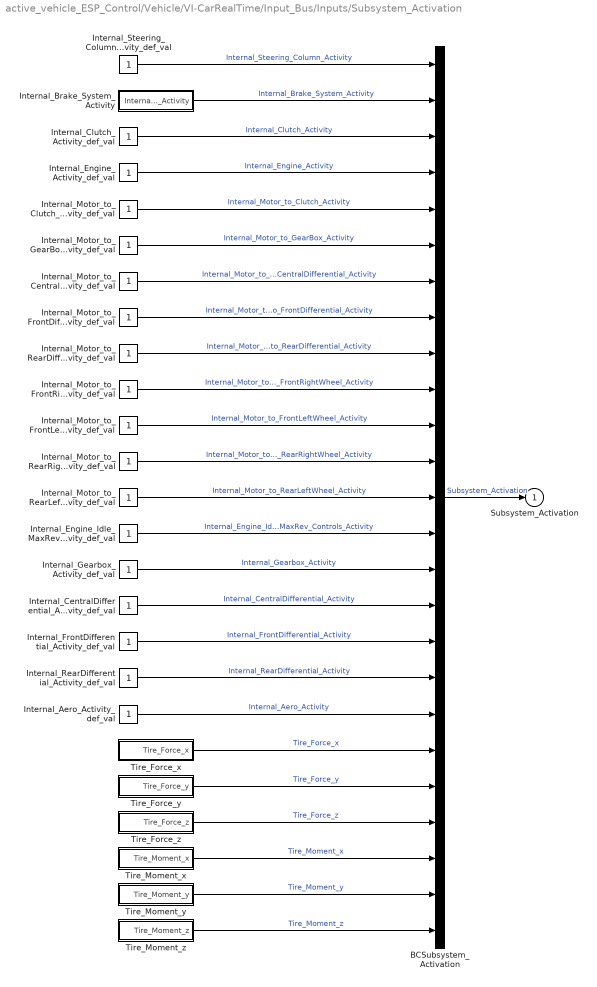
== system active_vehicle_ESP_Control/Vehicle/VI-CarRealTime/Input_Bus/Inputs/Subsystem_Activation ==
  BCSubsystem_Activation : BusCreator  Inputs=25
  Internal_Aero_Activity_def_val : Constant
  Internal_Brake_System_Activity : Subsystem
  Internal_CentralDifferential_Activity_def_val : Constant
  Internal_Clutch_Activity_def_val : Constant
  Internal_Engine_Activity_def_val : Constant
  Internal_Engine_Idle_MaxRev_Controls_Activity_def_val : Constant
  Internal_FrontDifferential_Activity_def_val : Constant
  Internal_Gearbox_Activity_def_val : Constant
  Internal_Motor_to_CentralDifferential_Activity_def_val : Constant
  Internal_Motor_to_Clutch_Activity_def_val : Constant
  Internal_Motor_to_FrontDifferential_Activity_def_val : Constant
  Internal_Motor_to_FrontLeftWheel_Activity_def_val : Constant
  Internal_Motor_to_FrontRightWheel_Activity_def_val : Constant
  Internal_Motor_to_GearBox_Activity_def_val : Constant
  Internal_Motor_to_RearDifferential_Activity_def_val : Constant
  Internal_Motor_to_RearLeftWheel_Activity_def_val : Constant
  Internal_Motor_to_RearRightWheel_Activity_def_val : Constant
  Internal_RearDifferential_Activity_def_val : Constant
  Internal_Steering_Column_Activity_def_val : Constant
  Tire_Force_x : Subsystem
  Tire_Force_y : Subsystem
  Tire_Force_z : Subsystem
  Tire_Moment_x : Subsystem
  Tire_Moment_y : Subsystem
  Tire_Moment_z : Subsystem
  Subsystem_Activation : Outport
  wires:
  BCSubsystem_Activation/1 -> Subsystem_Activation/1  "Subsystem_Activation"
  Internal_Steering_Column_Activity_def_val/1 -> BCSubsystem_Activation/1  "Internal_Steering_Column_Activity"
  Internal_Brake_System_Activity/1(Internal_Brake_System_Activity) -> BCSubsystem_Activation/2  "Internal_Brake_System_Activity"
  Internal_Clutch_Activity_def_val/1 -> BCSubsystem_Activation/3  "Internal_Clutch_Activity"
  Internal_Engine_Activity_def_val/1 -> BCSubsystem_Activation/4  "Internal_Engine_Activity"
  Internal_Motor_to_Clutch_Activity_def_val/1 -> BCSubsystem_Activation/5  "Internal_Motor_to_Clutch_Activity"
  Internal_Motor_to_GearBox_Activity_def_val/1 -> BCSubsystem_Activation/6  "Internal_Motor_to_GearBox_Activity"
  Internal_Motor_to_CentralDifferential_Activity_def_val/1 -> BCSubsystem_Activation/7  "Internal_Motor_to_CentralDifferential_Activity"
  Internal_Motor_to_FrontDifferential_Activity_def_val/1 -> BCSubsystem_Activation/8  "Internal_Motor_to_FrontDifferential_Activity"
  Internal_Motor_to_RearDifferential_Activity_def_val/1 -> BCSubsystem_Activation/9  "Internal_Motor_to_RearDifferential_Activity"
  Internal_Motor_to_FrontRightWheel_Activity_def_val/1 -> BCSubsystem_Activation/10  "Internal_Motor_to_FrontRightWheel_Activity"
  Internal_Motor_to_FrontLeftWheel_Activity_def_val/1 -> BCSubsystem_Activation/11  "Internal_Motor_to_FrontLeftWheel_Activity"
  Internal_Motor_to_RearRightWheel_Activity_def_val/1 -> BCSubsystem_Activation/12  "Internal_Motor_to_RearRightWheel_Activity"
  Internal_Motor_to_RearLeftWheel_Activity_def_val/1 -> BCSubsystem_Activation/13  "Internal_Motor_to_RearLeftWheel_Activity"
  Internal_Engine_Idle_MaxRev_Controls_Activity_def_val/1 -> BCSubsystem_Activation/14  "Internal_Engine_Idle_MaxRev_Controls_Activity"
  Internal_Gearbox_Activity_def_val/1 -> BCSubsystem_Activation/15  "Internal_Gearbox_Activity"
  Internal_CentralDifferential_Activity_def_val/1 -> BCSubsystem_Activation/16  "Internal_CentralDifferential_Activity"
  Internal_FrontDifferential_Activity_def_val/1 -> BCSubsystem_Activation/17  "Internal_FrontDifferential_Activity"
  Internal_RearDifferential_Activity_def_val/1 -> BCSubsystem_Activation/18  "Internal_RearDifferential_Activity"
  Internal_Aero_Activity_def_val/1 -> BCSubsystem_Activation/19  "Internal_Aero_Activity"
  Tire_Force_x/1(Tire_Force_x) -> BCSubsystem_Activation/20  "Tire_Force_x"
  Tire_Force_y/1(Tire_Force_y) -> BCSubsystem_Activation/21  "Tire_Force_y"
  Tire_Force_z/1(Tire_Force_z) -> BCSubsystem_Activation/22  "Tire_Force_z"
  Tire_Moment_x/1(Tire_Moment_x) -> BCSubsystem_Activation/23  "Tire_Moment_x"
  Tire_Moment_y/1(Tire_Moment_y) -> BCSubsystem_Activation/24  "Tire_Moment_y"
  Tire_Moment_z/1(Tire_Moment_z) -> BCSubsystem_Activation/25  "Tire_Moment_z"

== system active_vehicle_ESP_Control/Vehicle/VI-CarRealTime/Input_Bus/Inputs/TCS ==
  BCTCS : BusCreator  Inputs=2
  Internal_TCS_Activity_def_val : Constant
  TCS_threshold_def_val : Constant  Value=0
  TCS : Outport
  wires:
  BCTCS/1 -> TCS/1  "TCS"
  Internal_TCS_Activity_def_val/1 -> BCTCS/1  "Internal_TCS_Activity"
  TCS_threshold_def_val/1 -> BCTCS/2  "TCS_threshold"

== system active_vehicle_ESP_Control/Vehicle/VI-CarRealTime/Input_Bus/Inputs/Third_Element ==
  BCThird_Element : BusCreator  Inputs=4
  Damper_activity_flag : Subsystem
  Damper_force : Subsystem
  Spring : Subsystem
  Spring_activity_flag : Subsystem
  Third_Element : Outport
  wires:
  BCThird_Element/1 -> Third_Element/1  "Third_Element"
  Damper_force/1(Damper_force) -> BCThird_Element/1  "Damper_force"
  Damper_activity_flag/1(Damper_activity_flag) -> BCThird_Element/2  "Damper_activity_flag"
  Spring/1(Spring) -> BCThird_Element/3  "Spring"
  Spring_activity_flag/1(Spring_activity_flag) -> BCThird_Element/4  "Spring_activity_flag"

== system active_vehicle_ESP_Control/Vehicle/VI-CarRealTime/Input_Bus/Inputs/Tire_Force ==
  BCTire_Force : BusCreator  Inputs=3
  Fx : Subsystem
  Fy : Subsystem
  Fz : Subsystem
  Tire_Force : Outport
  wires:
  BCTire_Force/1 -> Tire_Force/1  "Tire_Force"
  Fx/1(Fx) -> BCTire_Force/1  "Fx"
  Fy/1(Fy) -> BCTire_Force/2  "Fy"
  Fz/1(Fz) -> BCTire_Force/3  "Fz"

== system active_vehicle_ESP_Control/Vehicle/VI-CarRealTime/Input_Bus/Inputs/Tire_Moment ==
  BCTire_Moment : BusCreator  Inputs=3
  Mx : Subsystem
  My : Subsystem
  Mz : Subsystem
  Tire_Moment : Outport
  wires:
  BCTire_Moment/1 -> Tire_Moment/1  "Tire_Moment"
  Mx/1(Mx) -> BCTire_Moment/1  "Mx"
  My/1(My) -> BCTire_Moment/2  "My"
  Mz/1(Mz) -> BCTire_Moment/3  "Mz"

== system active_vehicle_ESP_Control/Vehicle/VI-CarRealTime/Input_Bus/Inputs/Wheel_driving ==
  BCWheel_driving : BusCreator  Inputs=1
  moment : Subsystem
  Wheel_driving : Outport
  wires:
  BCWheel_driving/1 -> Wheel_driving/1  "Wheel_driving"
  moment/1(moment) -> BCWheel_driving/1  "moment"

== system active_vehicle_ESP_Control/Vehicle/VI-CarRealTime/Input_Bus/Inputs/Antiroll_Bar/activity_flag ==
  BCactivity_flag : BusCreator  Inputs=2
  front_def_val : Constant
  rear_def_val : Constant
  activity_flag : Outport
  wires:
  BCactivity_flag/1 -> activity_flag/1  "activity_flag"
  front_def_val/1 -> BCactivity_flag/1  "front"
  rear_def_val/1 -> BCactivity_flag/2  "rear"

== system active_vehicle_ESP_Control/Vehicle/VI-CarRealTime/Input_Bus/Inputs/Antiroll_Bar/force ==
  BCforce : BusCreator  Inputs=2
  front_def_val : Constant  Value=0
  rear_def_val : Constant  Value=0
  force : Outport
  wires:
  BCforce/1 -> force/1  "force"
  front_def_val/1 -> BCforce/1  "front"
  rear_def_val/1 -> BCforce/2  "rear"

== system active_vehicle_ESP_Control/Vehicle/VI-CarRealTime/Input_Bus/Inputs/Auxiliary_vertical/activity_flag ==
  BCactivity_flag : BusCreator  Inputs=4
  L1_def_val : Constant
  L2_def_val : Constant
  R1_def_val : Constant
  R2_def_val : Constant
  activity_flag : Outport
  wires:
  BCactivity_flag/1 -> activity_flag/1  "activity_flag"
  L1_def_val/1 -> BCactivity_flag/1  "L1"
  L2_def_val/1 -> BCactivity_flag/2  "L2"
  R1_def_val/1 -> BCactivity_flag/3  "R1"
  R2_def_val/1 -> BCactivity_flag/4  "R2"

== system active_vehicle_ESP_Control/Vehicle/VI-CarRealTime/Input_Bus/Inputs/Auxiliary_vertical/force ==
  BCforce : BusCreator  Inputs=4
  L1_def_val : Constant  Value=0
  L2_def_val : Constant  Value=0
  R1_def_val : Constant  Value=0
  R2_def_val : Constant  Value=0
  force : Outport
  wires:
  BCforce/1 -> force/1  "force"
  L1_def_val/1 -> BCforce/1  "L1"
  L2_def_val/1 -> BCforce/2  "L2"
  R1_def_val/1 -> BCforce/3  "R1"
  R2_def_val/1 -> BCforce/4  "R2"

== system active_vehicle_ESP_Control/Vehicle/VI-CarRealTime/Input_Bus/Inputs/Brake_System/brk_mmag_sign ==
  BCbrk_mmag_sign : BusCreator  Inputs=4
  L1_def_val : Constant  Value=0
  L2_def_val : Constant  Value=0
  R1_def_val : Constant  Value=0
  R2_def_val : Constant  Value=0
  brk_mmag_sign : Outport
  wires:
  BCbrk_mmag_sign/1 -> brk_mmag_sign/1  "brk_mmag_sign"
  L1_def_val/1 -> BCbrk_mmag_sign/1  "L1"
  L2_def_val/1 -> BCbrk_mmag_sign/2  "L2"
  R1_def_val/1 -> BCbrk_mmag_sign/3  "R1"
  R2_def_val/1 -> BCbrk_mmag_sign/4  "R2"

== system active_vehicle_ESP_Control/Vehicle/VI-CarRealTime/Input_Bus/Inputs/Brake_System/brk_mmag_unsign ==
  BCbrk_mmag_unsign : BusCreator  Inputs=4
  L1_def_val : Constant  Value=0
  L2_def_val : Constant  Value=0
  R1_def_val : Constant  Value=0
  R2_def_val : Constant  Value=0
  brk_mmag_unsign : Outport
  wires:
  BCbrk_mmag_unsign/1 -> brk_mmag_unsign/1  "brk_mmag_unsign"
  L1_def_val/1 -> BCbrk_mmag_unsign/1  "L1"
  L2_def_val/1 -> BCbrk_mmag_unsign/2  "L2"
  R1_def_val/1 -> BCbrk_mmag_unsign/3  "R1"
  R2_def_val/1 -> BCbrk_mmag_unsign/4  "R2"

== system active_vehicle_ESP_Control/Vehicle/VI-CarRealTime/Input_Bus/Inputs/Brake_System/brk_mu ==
  BCbrk_mu : BusCreator  Inputs=4
  L1_def_val : Constant  Value=0
  L2_def_val : Constant  Value=0
  R1_def_val : Constant  Value=0
  R2_def_val : Constant  Value=0
  brk_mu : Outport
  wires:
  BCbrk_mu/1 -> brk_mu/1  "brk_mu"
  L1_def_val/1 -> BCbrk_mu/1  "L1"
  L2_def_val/1 -> BCbrk_mu/2  "L2"
  R1_def_val/1 -> BCbrk_mu/3  "R1"
  R2_def_val/1 -> BCbrk_mu/4  "R2"

== system active_vehicle_ESP_Control/Vehicle/VI-CarRealTime/Input_Bus/Inputs/Brake_System/brk_pres ==
  BCbrk_pres : BusCreator  Inputs=4
  L1_def_val : Constant  Value=0
  L2_def_val : Constant  Value=0
  R1_def_val : Constant  Value=0
  R2_def_val : Constant  Value=0
  brk_pres : Outport
  wires:
  BCbrk_pres/1 -> brk_pres/1  "brk_pres"
  L1_def_val/1 -> BCbrk_pres/1  "L1"
  L2_def_val/1 -> BCbrk_pres/2  "L2"
  R1_def_val/1 -> BCbrk_pres/3  "R1"
  R2_def_val/1 -> BCbrk_pres/4  "R2"

== system active_vehicle_ESP_Control/Vehicle/VI-CarRealTime/Input_Bus/Inputs/Brake_System/brk_pres_gain ==
  BCbrk_pres_gain : BusCreator  Inputs=4
  L1_def_val : Constant
  L2_def_val : Constant
  R1_def_val : Constant
  R2_def_val : Constant
  brk_pres_gain : Outport
  wires:
  BCbrk_pres_gain/1 -> brk_pres_gain/1  "brk_pres_gain"
  L1_def_val/1 -> BCbrk_pres_gain/1  "L1"
  L2_def_val/1 -> BCbrk_pres_gain/2  "L2"
  R1_def_val/1 -> BCbrk_pres_gain/3  "R1"
  R2_def_val/1 -> BCbrk_pres_gain/4  "R2"

== system active_vehicle_ESP_Control/Vehicle/VI-CarRealTime/Input_Bus/Inputs/Ext_Body/force ==
  BCforce : BusCreator  Inputs=3
  X_def_val : Constant  Value=0
  Y_def_val : Constant  Value=0
  Z_def_val : Constant  Value=0
  force : Outport
  wires:
  BCforce/1 -> force/1  "force"
  X_def_val/1 -> BCforce/1  "X"
  Y_def_val/1 -> BCforce/2  "Y"
  Z_def_val/1 -> BCforce/3  "Z"

== system active_vehicle_ESP_Control/Vehicle/VI-CarRealTime/Input_Bus/Inputs/Ext_Body/moment ==
  BCmoment : BusCreator  Inputs=3
  X_def_val : Constant  Value=0
  Y_def_val : Constant  Value=0
  Z_def_val : Constant  Value=0
  moment : Outport
  wires:
  BCmoment/1 -> moment/1  "moment"
  X_def_val/1 -> BCmoment/1  "X"
  Y_def_val/1 -> BCmoment/2  "Y"
  Z_def_val/1 -> BCmoment/3  "Z"

== system active_vehicle_ESP_Control/Vehicle/VI-CarRealTime/Input_Bus/Inputs/Ext_Ground/force ==
  BCforce : BusCreator  Inputs=3
  X_def_val : Constant  Value=0
  Y_def_val : Constant  Value=0
  Z_def_val : Constant  Value=0
  force : Outport
  wires:
  BCforce/1 -> force/1  "force"
  X_def_val/1 -> BCforce/1  "X"
  Y_def_val/1 -> BCforce/2  "Y"
  Z_def_val/1 -> BCforce/3  "Z"

== system active_vehicle_ESP_Control/Vehicle/VI-CarRealTime/Input_Bus/Inputs/Ext_Ground/moment ==
  BCmoment : BusCreator  Inputs=3
  X_def_val : Constant  Value=0
  Y_def_val : Constant  Value=0
  Z_def_val : Constant  Value=0
  moment : Outport
  wires:
  BCmoment/1 -> moment/1  "moment"
  X_def_val/1 -> BCmoment/1  "X"
  Y_def_val/1 -> BCmoment/2  "Y"
  Z_def_val/1 -> BCmoment/3  "Z"

== system active_vehicle_ESP_Control/Vehicle/VI-CarRealTime/Input_Bus/Inputs/Ext_Tracking/force ==
  BCforce : BusCreator  Inputs=2
  X_def_val : Constant  Value=0
  Y_def_val : Constant  Value=0
  force : Outport
  wires:
  BCforce/1 -> force/1  "force"
  X_def_val/1 -> BCforce/1  "X"
  Y_def_val/1 -> BCforce/2  "Y"

== system active_vehicle_ESP_Control/Vehicle/VI-CarRealTime/Input_Bus/Inputs/Ext_Tracking/moment ==
  BCmoment : BusCreator  Inputs=2
  X_def_val : Constant  Value=0
  Y_def_val : Constant  Value=0
  moment : Outport
  wires:
  BCmoment/1 -> moment/1  "moment"
  X_def_val/1 -> BCmoment/1  "X"
  Y_def_val/1 -> BCmoment/2  "Y"

== system active_vehicle_ESP_Control/Vehicle/VI-CarRealTime/Input_Bus/Inputs/Friction/tire_mu ==
  BCtire_mu : BusCreator  Inputs=4
  L1_def_val : Constant  Value=0
  L2_def_val : Constant  Value=0
  R1_def_val : Constant  Value=0
  R2_def_val : Constant  Value=0
  tire_mu : Outport
  wires:
  BCtire_mu/1 -> tire_mu/1  "tire_mu"
  L1_def_val/1 -> BCtire_mu/1  "L1"
  L2_def_val/1 -> BCtire_mu/2  "L2"
  R1_def_val/1 -> BCtire_mu/3  "R1"
  R2_def_val/1 -> BCtire_mu/4  "R2"

== system active_vehicle_ESP_Control/Vehicle/VI-CarRealTime/Input_Bus/Inputs/Hook/Fx ==
  BCFx : BusCreator  Inputs=1
  rear_def_val : Constant  Value=0
  Fx : Outport
  wires:
  BCFx/1 -> Fx/1  "Fx"
  rear_def_val/1 -> BCFx/1  "rear"

== system active_vehicle_ESP_Control/Vehicle/VI-CarRealTime/Input_Bus/Inputs/Hook/Fy ==
  BCFy : BusCreator  Inputs=1
  rear_def_val : Constant  Value=0
  Fy : Outport
  wires:
  BCFy/1 -> Fy/1  "Fy"
  rear_def_val/1 -> BCFy/1  "rear"

== system active_vehicle_ESP_Control/Vehicle/VI-CarRealTime/Input_Bus/Inputs/Hook/Fz ==
  BCFz : BusCreator  Inputs=1
  rear_def_val : Constant  Value=0
  Fz : Outport
  wires:
  BCFz/1 -> Fz/1  "Fz"
  rear_def_val/1 -> BCFz/1  "rear"

== system active_vehicle_ESP_Control/Vehicle/VI-CarRealTime/Input_Bus/Inputs/Hook/Mx ==
  BCMx : BusCreator  Inputs=1
  rear_def_val : Constant  Value=0
  Mx : Outport
  wires:
  BCMx/1 -> Mx/1  "Mx"
  rear_def_val/1 -> BCMx/1  "rear"

== system active_vehicle_ESP_Control/Vehicle/VI-CarRealTime/Input_Bus/Inputs/Hook/My ==
  BCMy : BusCreator  Inputs=1
  rear_def_val : Constant  Value=0
  My : Outport
  wires:
  BCMy/1 -> My/1  "My"
  rear_def_val/1 -> BCMy/1  "rear"

== system active_vehicle_ESP_Control/Vehicle/VI-CarRealTime/Input_Bus/Inputs/Hook/Mz ==
  BCMz : BusCreator  Inputs=1
  rear_def_val : Constant  Value=0
  Mz : Outport
  wires:
  BCMz/1 -> Mz/1  "Mz"
  rear_def_val/1 -> BCMz/1  "rear"
